simulink model "Timestamp_delta_C_block_model"  (R2021b)
settings: Solver=FixedStepAuto  StartTime=0.0  StopTime=50  RelTol=1e-3
undefined symbols (not defined in the file): findUnixTime, input, T
settings Model: Creator=kilyovsk  LastModifiedBy=kilyovsk
settings SolverCC: ConcurrentTasks=on  PositivePriorityOrder=on
settings OptimizationCC: BlockReduction=off  OptimizeBlockIOStorage=off
settings DebuggingCC: TasksWithSamePriorityMsg=none
settings HardwareCC: ProdBitPerLong=64  ProdLongLongMode=on  ProdHWDeviceType=Intel->x86-64 (Linux 64)
settings SFSimCC: SimCustomHeaderCode=|
  | #include "getTime.h"
  | #include "findDelta.h"
settings SFSimCC: SimUserSources=|
  | getTime_script.c
  | findDelta_script.c
settings RTWCC: Description=Simulink Real-Time  SystemTargetFile=slrealtime.tlc  TemplateMakefile=slrealtime_default_tmf  Toolchain=Simulink Real-Time Toolchain  BuildConfiguration=Faster Runs  CodeExecutionProfiling=on  TargetLang=C++
settings RTWCC: CustomHeaderCode=|
  | #include "findDelta.h"
  | #include "getTime.h"
settings RTWCC: CustomSource=|
  | findDelta_script.c
  | getTime_script.c

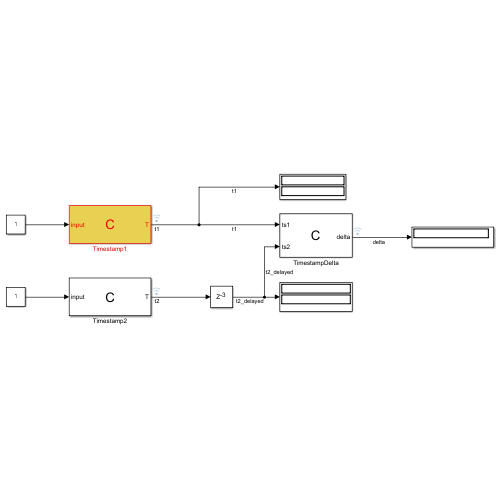
[thumbnail: Simulink's stored preview of the top-level diagram]
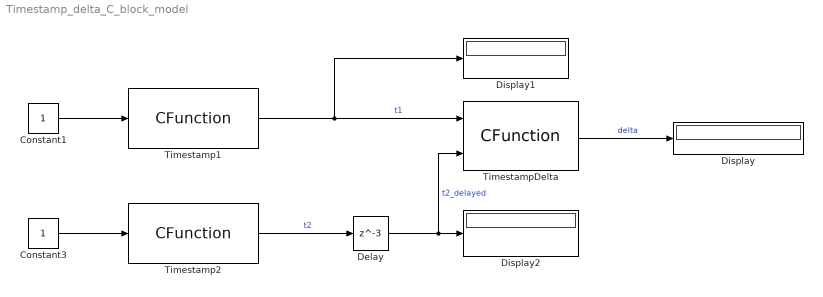
== system Timestamp_delta_C_block_model ==
  Constant1 : Constant
  Constant3 : Constant
  Delay : Delay  DelayLength=3  InitialCondition=0
  Display : Display
  Display1 : Display
  Display2 : Display
  Timestamp1 : CFunction  OutputCode=findUnixTime(T, input);
  Timestamp2 : CFunction  OutputCode=findUnixTime(T, input);
  TimestampDelta : CFunction  OutputCode=delta = findDelta(ts1, ts2);
  wires:
  Delay/1 -> Display2/1, TimestampDelta/2  "t2_delayed"
  Timestamp1/1 -> TimestampDelta/1, Display1/1  "t1"
  Timestamp2/1 -> Delay/1  "t2"
  TimestampDelta/1 -> Display/1  "delta"
  Constant1/1 -> Timestamp1/1
  Constant3/1 -> Timestamp2/1
